simulink model "DC_motor"  (R2023a)
settings: Solver=VariableStepAuto  StartTime=0.0  StopTime=1.0  RelTol=1e-3
model workspace: external: MATLAB File /Users/motya/School/2024/ТАУ/laba_1/config.m (data not in the file)
values from neighbouring files (symbols this model uses):
  b = 0.001    [config.m]
  C_m = 1.3    [config.m]
  C_w = 3.15    [config.m]
  J = 7 * 10^(-6)    (= 7e-06)    [config.m]
  L_a = 0.0015    [config.m]
  L_f = 0.013    [config.m]
  R_a = 8    [config.m]
settings Model: Creator=motya  LastModifiedBy=motya

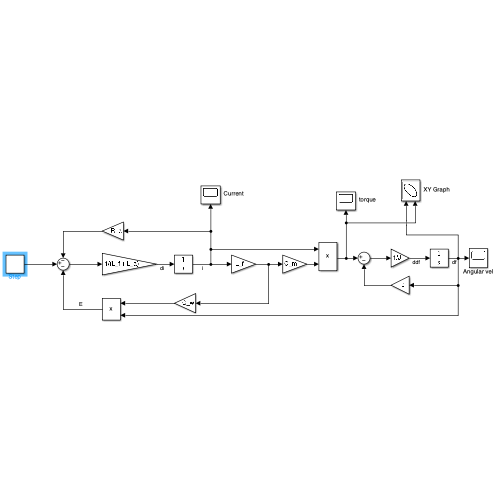
[thumbnail: Simulink's stored preview of the top-level diagram]
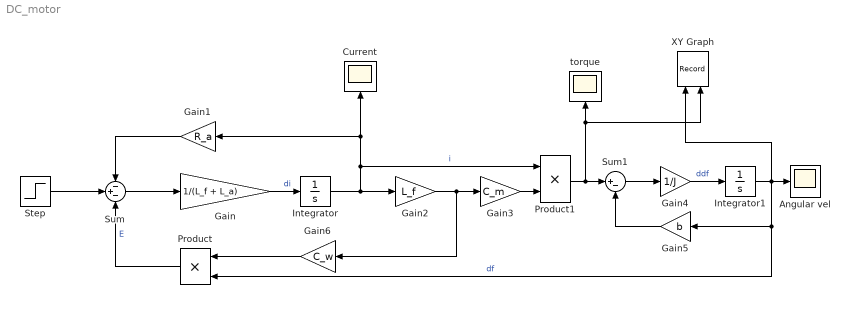
== system DC_motor ==
  Angular vel : Scope
  Current : Scope
  Gain : Gain  Gain=1/(L_f + L_a)
  Gain1 : Gain  Gain=R_a
  Gain2 : Gain  Gain=L_f
  Gain3 : Gain  Gain=C_m
  Gain4 : Gain  Gain=1/J
  Gain5 : Gain  Gain=b
  Gain6 : Gain  Gain=C_w
  Integrator : Integrator
  Integrator1 : Integrator
  Product : Product
  Product1 : Product
  Step : Step  Time=0  After=5  SampleTime=0
  Sum : Sum  Inputs=-+-
  Sum1 : Sum  Inputs=|+-
  XY Graph : Record  FileSettingsInternal="{\"entries\":[{\"content\":{\"excelSettings\":{\"content\":{},\"type\":\"Streamout.ExcelSettings\"}},\"type\":\"Streamout.FileSettingStorage\",\"uuid\":\"\"}],\"packageUris\":[\"http:\\/\\/schema.mathworks.com\\/mf0\\/streamout_blocks\\/R2020a\"],\"version\":\"1.0\"}"  Layout=[1 1]  SignalsInternal="{\"entries\":[{\"content\":{\"signals\":[{\"content\":{\"blockPath\":[],\"dimensions\":[1],\"domain\":\"\",\"lineColor\":\"#a2142f\",\"plots\":[1],\"port\":1,\"sid\":[\"\"],\"signalID\":103,\"signalName\":\"df\"},\"type\":\"RecordBlkView.Signal\",\"uuid\":\"\"},{\"content\":{\"blockPath\":[],\"dimensions\":[1],\"domain\":\"\",\"lineColor\":\"#139fff\",\"plots\":[1],\"port\":2,\"sid\":[\"\"],\"signalID\":107,\"signalName\":\"Product1\"},\"type\":\"RecordBlkView.Signal\",\"uuid\":\"\"}]},\"type\":\"RecordBlkView.InputSignals\",\"uuid\":\"\"}],\"packageUris\":[\"http:\\/\\/schema.mathworks.com\\/mf0\\/streamout_blocks\\/R2020a\"],\"version\":\"1.0\"}"  VisualizationBindings="{\"xyplotplugin\":{\"info\":[{\"series\":[{\"bindingParametersList\":[{\"parameter\":\"X-Axis\",\"signalID\":103,\"signalName\":\"df\"},{\"parameter\":\"Y-Axis\",\"signalID\":107,\"signalName\":\"Product1\"}],\"seriesID\":28749}],\"subplotID\":1}]}}"  CompatibilityTag=XY
  torque : Scope
  wires:
  Sum/1 -> Gain/1
  Integrator/1 -> Gain2/1, Current/1, Gain1/1, Product1/1  "i"
  Gain1/1 -> Sum/1
  Gain/1 -> Integrator/1  "di"
  Sum1/1 -> Gain4/1
  Gain4/1 -> Integrator1/1  "ddf"
  Integrator1/1 -> Angular vel/1, XY Graph/1, Product/2, Gain5/1  "df"
  Gain5/1 -> Sum1/2
  Gain2/1 -> Gain6/1, Gain3/1
  Step/1 -> Sum/2
  Gain3/1 -> Product1/2
  Product1/1 -> Sum1/1, torque/1, XY Graph/2
  Gain6/1 -> Product/1
  Product/1 -> Sum/3  "E"
